simulink model "ReactionWheel"  (R2020a)
settings: Solver=FixedStepAuto  StartTime=0.0  StopTime=100  FixedStep=0.00005  RelTol=1e-3
libraries: simulink x8, aerolibconvert2 x2
settings Model: Creator=b_ant  LastModifiedBy=DELL

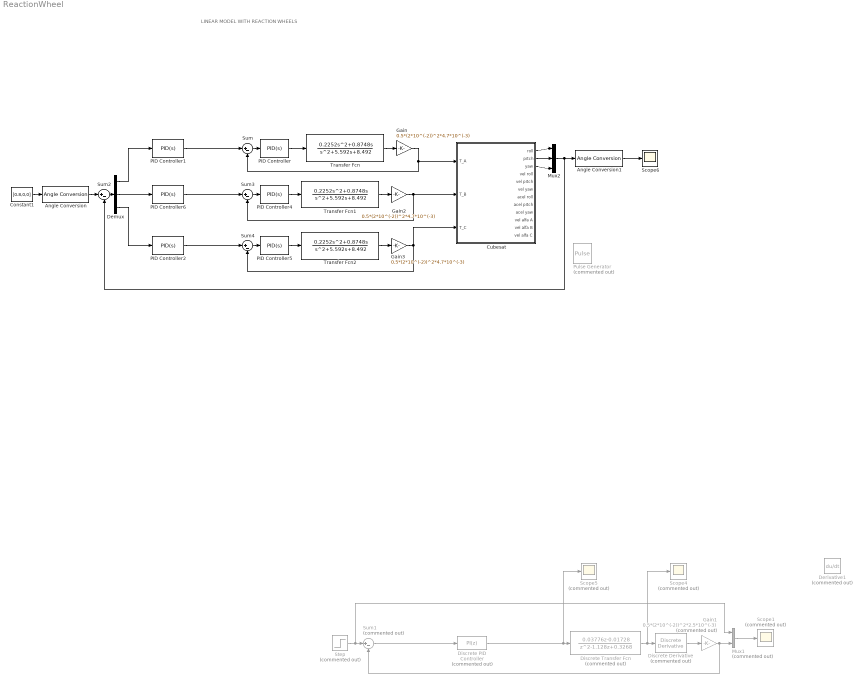
== system ReactionWheel ==
  note: LINEAR MODEL WITH REACTION WHEELS
  Angle Conversion : aerolibconvert2/Angle Conversion  IU=deg  OU=rad
  Angle Conversion1 : aerolibconvert2/Angle Conversion  IU=rad  OU=deg
  Constant1 : Constant  Value=[0.8,0,0]
  Cubesat : Subsystem  mask{Iw=9.4*10^-7, Ib=6.88*10^-4, mw=0.0047, lw=0.092, Bw=0}
      mask prompts: Iw "Momento de inercia de rueda de reacción"; Ib "Momento de inercia de CubeSat"; mw "Masa de Rueda de reacción"; lw "Longitud de CM de CubeSat a eje de rueda"; Bw "Coeficiente de friccion"
  Demux : Demux  Outputs=3
  Derivative1 : Derivative  Commented=on
  Discrete Transfer Fcn : DiscreteTransferFcn  Commented=on  Numerator=[0.03776 -0.01728]  Denominator=[1 -1.128 0.3268]
  Discrete Derivative : simulink/Discrete/Discrete Derivative  Commented=on  gainval=1  ICPrevScaledInput=0  OutMin=[]  OutMax=[]  OutDataType=fixdt(1, 16)  OutScaling=2^-10  DoSatur=off
  Discrete PID Controller : simulink/Continuous/PID Controller  Commented=on  Controller=PI  Form=Parallel  TimeDomain=Discrete-time  UseExternalTs=off  SampleTime=0.1  IntegratorMethod=Trapezoidal  FilterMethod=Forward Euler  ControllerParametersSource=internal  P=2275968.39507176  I=49240241.1330709  D=0  UseFilter=on  N=100  TunerSelectOption=Transfer Function Based (PID Tuner App)  InitialConditionSource=internal  InitialConditionForIntegrator=0  InitialConditionForFilter=0  DifferentiatorICPrevScaledInput=0  ExternalReset=none  TrackingMode=off  Kt=1  LimitOutput=on  UpperSaturationLimit=4999  LowerSaturationLimit=-4999  LinearizeAsGain=on  AntiWindupMode=none  Kb=1  POutMin=[]  POutMax=[]  IOutMin=[]  IOutMax=[]  DOutMin=[]  DOutMax=[]  NOutMin=[]  NOutMax=[]  SumOutMin=[]  SumOutMax=[]  SaturationOutMin=[]  SaturationOutMax=[]  PParamMin=[]  PParamMax=[]  IParamMin=[]  IParamMax=[]  DParamMin=[]  DParamMax=[]  NParamMin=[]  NParamMax=[]  KbParamMin=[]  KbParamMax=[]  KtParamMin=[]  KtParamMax=[]  KbOutMin=[]  KbOutMax=[]  KtOutMin=[]  KtOutMax=[]  IntegratorOutMin=[]  IntegratorOutMax=[]  FilterOutMin=[]  FilterOutMax=[]  SumI1OutMin=[]  SumI1OutMax=[]  SumI2OutMin=[]  SumI2OutMax=[]  SumI3OutMin=[]  SumI3OutMax=[]  SumI4OutMin=[]  SumI4OutMax=[]  SumDOutMin=[]  SumDOutMax=[]  DifferentiatorOutMin=[]  DifferentiatorOutMax=[]  FilterDiffOutCoefMin=[]  FilterDiffOutCoefMax=[]  ReciprocalOutMin=[]  ReciprocalOutMax=[]  SumDenOutMin=[]  SumDenOutMax=[]  SumNumOutMin=[]  SumNumOutMax=[]  DivideOutMin=[]  DivideOutMax=[]  UdiffTsProdOutMin=[]  UdiffTsProdOutMax=[]  NTsProdOutMin=[]  NTsProdOutMax=[]  UintegralTsProdOutMin=[]  UintegralTsProdOutMax=[]  UngainTsProdOutMin=[]  UngainTsProdOutMax=[]  IntegratorContinuousStateAttributes=''  IntegratorStateMustResolveToSignalObject=off  IntegratorRTWStateStorageClass=Auto  FilterContinuousStateAttributes=''  FilterStateMustResolveToSignalObject=off  FilterRTWStateStorageClass=Auto  ParallelPVariant=InternalParameters  IdealPVariant=Disabled  IVariant=InternalParameters  DVariant=Disabled  IntegratorVariant=Discrete  SatVariant=Enabled  AWVariant=Passthrough  PCopyVariant=Disabled  TRVariant=Disabled  FdbkBlocksVariant=Forward  IdealPFdbkVariant=Disabled  SatFdbkVariant=Disabled  DerivativeFilterVariant=Disabled  NVariant=Disabled  NCopyVariant=Disabled_SignalSpec  FilterICVariant=Disabled  IntegratorICVariant=InternalICs  ExternalResetVariant=Disabled  TRSumVariant=Passthrough  SumFdbkVariant=Disabled  SumVariant=Sum_PI  TsampFilterVariant=InternalTs  TsampNgainVariant=Passthrough  TsampIntegralVariant=Passthrough
  Gain : Gain  Gain=0.5*(2*10^(-2))^2*4.7*10^(-3)
  Gain1 : Gain  Commented=on  Gain=0.5*(2*10^(-2))^2*2.5*10^(-3)
  Gain2 : Gain  Gain=0.5*(2*10^(-2))^2*4.7*10^(-3)
  Gain3 : Gain  Gain=0.5*(2*10^(-2))^2*4.7*10^(-3)
  Mux1 : Mux  Commented=on  Inputs=2
  Mux2 : Mux  Inputs=3
  PID Controller : simulink/Continuous/PID Controller  Controller=PID  Form=Parallel  TimeDomain=Continuous-time  UseExternalTs=off  SampleTime=1  IntegratorMethod=Forward Euler  FilterMethod=Forward Euler  ControllerParametersSource=internal  P=0  I=15673894481.5576  D=0  UseFilter=on  N=100  TunerSelectOption=Transfer Function Based (PID Tuner App)  InitialConditionSource=internal  InitialConditionForIntegrator=0  InitialConditionForFilter=0  DifferentiatorICPrevScaledInput=0  ExternalReset=none  TrackingMode=off  Kt=1  LimitOutput=on  UpperSaturationLimit=4999  LowerSaturationLimit=-4999  LinearizeAsGain=on  AntiWindupMode=none  Kb=1  POutMin=[]  POutMax=[]  IOutMin=[]  IOutMax=[]  DOutMin=[]  DOutMax=[]  NOutMin=[]  NOutMax=[]  SumOutMin=[]  SumOutMax=[]  SaturationOutMin=[]  SaturationOutMax=[]  PParamMin=[]  PParamMax=[]  IParamMin=[]  IParamMax=[]  DParamMin=[]  DParamMax=[]  NParamMin=[]  NParamMax=[]  KbParamMin=[]  KbParamMax=[]  KtParamMin=[]  KtParamMax=[]  KbOutMin=[]  KbOutMax=[]  KtOutMin=[]  KtOutMax=[]  IntegratorOutMin=[]  IntegratorOutMax=[]  FilterOutMin=[]  FilterOutMax=[]  SumI1OutMin=[]  SumI1OutMax=[]  SumI2OutMin=[]  SumI2OutMax=[]  SumI3OutMin=[]  SumI3OutMax=[]  SumI4OutMin=[]  SumI4OutMax=[]  SumDOutMin=[]  SumDOutMax=[]  DifferentiatorOutMin=[]  DifferentiatorOutMax=[]  FilterDiffOutCoefMin=[]  FilterDiffOutCoefMax=[]  ReciprocalOutMin=[]  ReciprocalOutMax=[]  SumDenOutMin=[]  SumDenOutMax=[]  SumNumOutMin=[]  SumNumOutMax=[]  DivideOutMin=[]  DivideOutMax=[]  UdiffTsProdOutMin=[]  UdiffTsProdOutMax=[]  NTsProdOutMin=[]  NTsProdOutMax=[]  UintegralTsProdOutMin=[]  UintegralTsProdOutMax=[]  UngainTsProdOutMin=[]  UngainTsProdOutMax=[]  IntegratorContinuousStateAttributes=''  IntegratorStateMustResolveToSignalObject=off  IntegratorRTWStateStorageClass=Auto  FilterContinuousStateAttributes=''  FilterStateMustResolveToSignalObject=off  FilterRTWStateStorageClass=Auto  ParallelPVariant=InternalParameters  IdealPVariant=Disabled  IVariant=InternalParameters  DVariant=InternalParameters  IntegratorVariant=Continuous  SatVariant=Enabled  AWVariant=Passthrough  PCopyVariant=Disabled  TRVariant=Disabled  FdbkBlocksVariant=Forward  IdealPFdbkVariant=Disabled  SatFdbkVariant=Disabled  DerivativeFilterVariant=ContFilter  NVariant=InternalParameters  NCopyVariant=Disabled  FilterICVariant=InternalICsFilter  IntegratorICVariant=InternalICs  ExternalResetVariant=Disabled  TRSumVariant=Passthrough  SumFdbkVariant=Disabled  SumVariant=Sum_PID  TsampFilterVariant=InternalTs  TsampNgainVariant=Passthrough  TsampIntegralVariant=Passthrough
  PID Controller1 : simulink/Continuous/PID Controller  Controller=PID  Form=Parallel  TimeDomain=Continuous-time  UseExternalTs=off  SampleTime=-1  IntegratorMethod=Forward Euler  FilterMethod=Forward Euler  ControllerParametersSource=internal  P=-3.24987577526797e-07  I=-2.1955547593358e-10  D=-8.46467148788469e-05  UseFilter=on  N=11.428279760416  TunerSelectOption=Transfer Function Based (PID Tuner App)  InitialConditionSource=internal  InitialConditionForIntegrator=0  InitialConditionForFilter=0  DifferentiatorICPrevScaledInput=0  ExternalReset=none  TrackingMode=off  Kt=1  LimitOutput=off  UpperSaturationLimit=3*10^(-3)  LowerSaturationLimit=-3*10^(-3)  LinearizeAsGain=on  AntiWindupMode=none  Kb=1  POutMin=[]  POutMax=[]  IOutMin=[]  IOutMax=[]  DOutMin=[]  DOutMax=[]  NOutMin=[]  NOutMax=[]  SumOutMin=[]  SumOutMax=[]  SaturationOutMin=[]  SaturationOutMax=[]  PParamMin=[]  PParamMax=[]  IParamMin=[]  IParamMax=[]  DParamMin=[]  DParamMax=[]  NParamMin=[]  NParamMax=[]  KbParamMin=[]  KbParamMax=[]  KtParamMin=[]  KtParamMax=[]  KbOutMin=[]  KbOutMax=[]  KtOutMin=[]  KtOutMax=[]  IntegratorOutMin=[]  IntegratorOutMax=[]  FilterOutMin=[]  FilterOutMax=[]  SumI1OutMin=[]  SumI1OutMax=[]  SumI2OutMin=[]  SumI2OutMax=[]  SumI3OutMin=[]  SumI3OutMax=[]  SumI4OutMin=[]  SumI4OutMax=[]  SumDOutMin=[]  SumDOutMax=[]  DifferentiatorOutMin=[]  DifferentiatorOutMax=[]  FilterDiffOutCoefMin=[]  FilterDiffOutCoefMax=[]  ReciprocalOutMin=[]  ReciprocalOutMax=[]  SumDenOutMin=[]  SumDenOutMax=[]  SumNumOutMin=[]  SumNumOutMax=[]  DivideOutMin=[]  DivideOutMax=[]  UdiffTsProdOutMin=[]  UdiffTsProdOutMax=[]  NTsProdOutMin=[]  NTsProdOutMax=[]  UintegralTsProdOutMin=[]  UintegralTsProdOutMax=[]  UngainTsProdOutMin=[]  UngainTsProdOutMax=[]  IntegratorContinuousStateAttributes=''  IntegratorStateMustResolveToSignalObject=off  IntegratorRTWStateStorageClass=Auto  FilterContinuousStateAttributes=''  FilterStateMustResolveToSignalObject=off  FilterRTWStateStorageClass=Auto  ParallelPVariant=InternalParameters  IdealPVariant=Disabled  IVariant=InternalParameters  DVariant=InternalParameters  IntegratorVariant=Continuous  SatVariant=Disabled  AWVariant=Passthrough  PCopyVariant=Disabled  TRVariant=Disabled  FdbkBlocksVariant=Forward  IdealPFdbkVariant=Disabled  SatFdbkVariant=Disabled  DerivativeFilterVariant=ContFilter  NVariant=InternalParameters  NCopyVariant=Disabled  FilterICVariant=InternalICsFilter  IntegratorICVariant=InternalICs  ExternalResetVariant=Disabled  TRSumVariant=Passthrough  SumFdbkVariant=Disabled  SumVariant=Sum_PID  TsampFilterVariant=InternalTs  TsampNgainVariant=Passthrough  TsampIntegralVariant=Passthrough
  PID Controller2 : simulink/Continuous/PID Controller  Controller=PID  Form=Parallel  TimeDomain=Continuous-time  UseExternalTs=off  SampleTime=-1  IntegratorMethod=Forward Euler  FilterMethod=Forward Euler  ControllerParametersSource=internal  P=-3.24987577526797e-07  I=-2.1955547593358e-10  D=-8.46467148788469e-05  UseFilter=on  N=11.428279760416  TunerSelectOption=Transfer Function Based (PID Tuner App)  InitialConditionSource=internal  InitialConditionForIntegrator=0  InitialConditionForFilter=0  DifferentiatorICPrevScaledInput=0  ExternalReset=none  TrackingMode=off  Kt=1  LimitOutput=off  UpperSaturationLimit=3*10^(-3)  LowerSaturationLimit=-3*10^(-3)  LinearizeAsGain=on  AntiWindupMode=none  Kb=1  POutMin=[]  POutMax=[]  IOutMin=[]  IOutMax=[]  DOutMin=[]  DOutMax=[]  NOutMin=[]  NOutMax=[]  SumOutMin=[]  SumOutMax=[]  SaturationOutMin=[]  SaturationOutMax=[]  PParamMin=[]  PParamMax=[]  IParamMin=[]  IParamMax=[]  DParamMin=[]  DParamMax=[]  NParamMin=[]  NParamMax=[]  KbParamMin=[]  KbParamMax=[]  KtParamMin=[]  KtParamMax=[]  KbOutMin=[]  KbOutMax=[]  KtOutMin=[]  KtOutMax=[]  IntegratorOutMin=[]  IntegratorOutMax=[]  FilterOutMin=[]  FilterOutMax=[]  SumI1OutMin=[]  SumI1OutMax=[]  SumI2OutMin=[]  SumI2OutMax=[]  SumI3OutMin=[]  SumI3OutMax=[]  SumI4OutMin=[]  SumI4OutMax=[]  SumDOutMin=[]  SumDOutMax=[]  DifferentiatorOutMin=[]  DifferentiatorOutMax=[]  FilterDiffOutCoefMin=[]  FilterDiffOutCoefMax=[]  ReciprocalOutMin=[]  ReciprocalOutMax=[]  SumDenOutMin=[]  SumDenOutMax=[]  SumNumOutMin=[]  SumNumOutMax=[]  DivideOutMin=[]  DivideOutMax=[]  UdiffTsProdOutMin=[]  UdiffTsProdOutMax=[]  NTsProdOutMin=[]  NTsProdOutMax=[]  UintegralTsProdOutMin=[]  UintegralTsProdOutMax=[]  UngainTsProdOutMin=[]  UngainTsProdOutMax=[]  IntegratorContinuousStateAttributes=''  IntegratorStateMustResolveToSignalObject=off  IntegratorRTWStateStorageClass=Auto  FilterContinuousStateAttributes=''  FilterStateMustResolveToSignalObject=off  FilterRTWStateStorageClass=Auto  ParallelPVariant=InternalParameters  IdealPVariant=Disabled  IVariant=InternalParameters  DVariant=InternalParameters  IntegratorVariant=Continuous  SatVariant=Disabled  AWVariant=Passthrough  PCopyVariant=Disabled  TRVariant=Disabled  FdbkBlocksVariant=Forward  IdealPFdbkVariant=Disabled  SatFdbkVariant=Disabled  DerivativeFilterVariant=ContFilter  NVariant=InternalParameters  NCopyVariant=Disabled  FilterICVariant=InternalICsFilter  IntegratorICVariant=InternalICs  ExternalResetVariant=Disabled  TRSumVariant=Passthrough  SumFdbkVariant=Disabled  SumVariant=Sum_PID  TsampFilterVariant=InternalTs  TsampNgainVariant=Passthrough  TsampIntegralVariant=Passthrough
  PID Controller4 : simulink/Continuous/PID Controller  Controller=PID  Form=Parallel  TimeDomain=Continuous-time  UseExternalTs=off  SampleTime=1  IntegratorMethod=Forward Euler  FilterMethod=Forward Euler  ControllerParametersSource=internal  P=0  I=15673894481.5576  D=0  UseFilter=on  N=100  TunerSelectOption=Transfer Function Based (PID Tuner App)  InitialConditionSource=internal  InitialConditionForIntegrator=0  InitialConditionForFilter=0  DifferentiatorICPrevScaledInput=0  ExternalReset=none  TrackingMode=off  Kt=1  LimitOutput=on  UpperSaturationLimit=4999  LowerSaturationLimit=-4999  LinearizeAsGain=on  AntiWindupMode=none  Kb=1  POutMin=[]  POutMax=[]  IOutMin=[]  IOutMax=[]  DOutMin=[]  DOutMax=[]  NOutMin=[]  NOutMax=[]  SumOutMin=[]  SumOutMax=[]  SaturationOutMin=[]  SaturationOutMax=[]  PParamMin=[]  PParamMax=[]  IParamMin=[]  IParamMax=[]  DParamMin=[]  DParamMax=[]  NParamMin=[]  NParamMax=[]  KbParamMin=[]  KbParamMax=[]  KtParamMin=[]  KtParamMax=[]  KbOutMin=[]  KbOutMax=[]  KtOutMin=[]  KtOutMax=[]  IntegratorOutMin=[]  IntegratorOutMax=[]  FilterOutMin=[]  FilterOutMax=[]  SumI1OutMin=[]  SumI1OutMax=[]  SumI2OutMin=[]  SumI2OutMax=[]  SumI3OutMin=[]  SumI3OutMax=[]  SumI4OutMin=[]  SumI4OutMax=[]  SumDOutMin=[]  SumDOutMax=[]  DifferentiatorOutMin=[]  DifferentiatorOutMax=[]  FilterDiffOutCoefMin=[]  FilterDiffOutCoefMax=[]  ReciprocalOutMin=[]  ReciprocalOutMax=[]  SumDenOutMin=[]  SumDenOutMax=[]  SumNumOutMin=[]  SumNumOutMax=[]  DivideOutMin=[]  DivideOutMax=[]  UdiffTsProdOutMin=[]  UdiffTsProdOutMax=[]  NTsProdOutMin=[]  NTsProdOutMax=[]  UintegralTsProdOutMin=[]  UintegralTsProdOutMax=[]  UngainTsProdOutMin=[]  UngainTsProdOutMax=[]  IntegratorContinuousStateAttributes=''  IntegratorStateMustResolveToSignalObject=off  IntegratorRTWStateStorageClass=Auto  FilterContinuousStateAttributes=''  FilterStateMustResolveToSignalObject=off  FilterRTWStateStorageClass=Auto  ParallelPVariant=InternalParameters  IdealPVariant=Disabled  IVariant=InternalParameters  DVariant=InternalParameters  IntegratorVariant=Continuous  SatVariant=Enabled  AWVariant=Passthrough  PCopyVariant=Disabled  TRVariant=Disabled  FdbkBlocksVariant=Forward  IdealPFdbkVariant=Disabled  SatFdbkVariant=Disabled  DerivativeFilterVariant=ContFilter  NVariant=InternalParameters  NCopyVariant=Disabled  FilterICVariant=InternalICsFilter  IntegratorICVariant=InternalICs  ExternalResetVariant=Disabled  TRSumVariant=Passthrough  SumFdbkVariant=Disabled  SumVariant=Sum_PID  TsampFilterVariant=InternalTs  TsampNgainVariant=Passthrough  TsampIntegralVariant=Passthrough
  PID Controller5 : simulink/Continuous/PID Controller  Controller=PID  Form=Parallel  TimeDomain=Continuous-time  UseExternalTs=off  SampleTime=1  IntegratorMethod=Forward Euler  FilterMethod=Forward Euler  ControllerParametersSource=internal  P=0  I=15673894481.5576  D=0  UseFilter=on  N=100  TunerSelectOption=Transfer Function Based (PID Tuner App)  InitialConditionSource=internal  InitialConditionForIntegrator=0  InitialConditionForFilter=0  DifferentiatorICPrevScaledInput=0  ExternalReset=none  TrackingMode=off  Kt=1  LimitOutput=on  UpperSaturationLimit=4999  LowerSaturationLimit=-4999  LinearizeAsGain=on  AntiWindupMode=none  Kb=1  POutMin=[]  POutMax=[]  IOutMin=[]  IOutMax=[]  DOutMin=[]  DOutMax=[]  NOutMin=[]  NOutMax=[]  SumOutMin=[]  SumOutMax=[]  SaturationOutMin=[]  SaturationOutMax=[]  PParamMin=[]  PParamMax=[]  IParamMin=[]  IParamMax=[]  DParamMin=[]  DParamMax=[]  NParamMin=[]  NParamMax=[]  KbParamMin=[]  KbParamMax=[]  KtParamMin=[]  KtParamMax=[]  KbOutMin=[]  KbOutMax=[]  KtOutMin=[]  KtOutMax=[]  IntegratorOutMin=[]  IntegratorOutMax=[]  FilterOutMin=[]  FilterOutMax=[]  SumI1OutMin=[]  SumI1OutMax=[]  SumI2OutMin=[]  SumI2OutMax=[]  SumI3OutMin=[]  SumI3OutMax=[]  SumI4OutMin=[]  SumI4OutMax=[]  SumDOutMin=[]  SumDOutMax=[]  DifferentiatorOutMin=[]  DifferentiatorOutMax=[]  FilterDiffOutCoefMin=[]  FilterDiffOutCoefMax=[]  ReciprocalOutMin=[]  ReciprocalOutMax=[]  SumDenOutMin=[]  SumDenOutMax=[]  SumNumOutMin=[]  SumNumOutMax=[]  DivideOutMin=[]  DivideOutMax=[]  UdiffTsProdOutMin=[]  UdiffTsProdOutMax=[]  NTsProdOutMin=[]  NTsProdOutMax=[]  UintegralTsProdOutMin=[]  UintegralTsProdOutMax=[]  UngainTsProdOutMin=[]  UngainTsProdOutMax=[]  IntegratorContinuousStateAttributes=''  IntegratorStateMustResolveToSignalObject=off  IntegratorRTWStateStorageClass=Auto  FilterContinuousStateAttributes=''  FilterStateMustResolveToSignalObject=off  FilterRTWStateStorageClass=Auto  ParallelPVariant=InternalParameters  IdealPVariant=Disabled  IVariant=InternalParameters  DVariant=InternalParameters  IntegratorVariant=Continuous  SatVariant=Enabled  AWVariant=Passthrough  PCopyVariant=Disabled  TRVariant=Disabled  FdbkBlocksVariant=Forward  IdealPFdbkVariant=Disabled  SatFdbkVariant=Disabled  DerivativeFilterVariant=ContFilter  NVariant=InternalParameters  NCopyVariant=Disabled  FilterICVariant=InternalICsFilter  IntegratorICVariant=InternalICs  ExternalResetVariant=Disabled  TRSumVariant=Passthrough  SumFdbkVariant=Disabled  SumVariant=Sum_PID  TsampFilterVariant=InternalTs  TsampNgainVariant=Passthrough  TsampIntegralVariant=Passthrough
  PID Controller6 : simulink/Continuous/PID Controller  Controller=PID  Form=Parallel  TimeDomain=Continuous-time  UseExternalTs=off  SampleTime=-1  IntegratorMethod=Forward Euler  FilterMethod=Forward Euler  ControllerParametersSource=internal  P=-3.24987577526797e-07  I=-2.1955547593358e-10  D=-8.46467148788469e-05  UseFilter=on  N=11.428279760416  TunerSelectOption=Transfer Function Based (PID Tuner App)  InitialConditionSource=internal  InitialConditionForIntegrator=0  InitialConditionForFilter=0  DifferentiatorICPrevScaledInput=0  ExternalReset=none  TrackingMode=off  Kt=1  LimitOutput=off  UpperSaturationLimit=3*10^(-3)  LowerSaturationLimit=-3*10^(-3)  LinearizeAsGain=on  AntiWindupMode=none  Kb=1  POutMin=[]  POutMax=[]  IOutMin=[]  IOutMax=[]  DOutMin=[]  DOutMax=[]  NOutMin=[]  NOutMax=[]  SumOutMin=[]  SumOutMax=[]  SaturationOutMin=[]  SaturationOutMax=[]  PParamMin=[]  PParamMax=[]  IParamMin=[]  IParamMax=[]  DParamMin=[]  DParamMax=[]  NParamMin=[]  NParamMax=[]  KbParamMin=[]  KbParamMax=[]  KtParamMin=[]  KtParamMax=[]  KbOutMin=[]  KbOutMax=[]  KtOutMin=[]  KtOutMax=[]  IntegratorOutMin=[]  IntegratorOutMax=[]  FilterOutMin=[]  FilterOutMax=[]  SumI1OutMin=[]  SumI1OutMax=[]  SumI2OutMin=[]  SumI2OutMax=[]  SumI3OutMin=[]  SumI3OutMax=[]  SumI4OutMin=[]  SumI4OutMax=[]  SumDOutMin=[]  SumDOutMax=[]  DifferentiatorOutMin=[]  DifferentiatorOutMax=[]  FilterDiffOutCoefMin=[]  FilterDiffOutCoefMax=[]  ReciprocalOutMin=[]  ReciprocalOutMax=[]  SumDenOutMin=[]  SumDenOutMax=[]  SumNumOutMin=[]  SumNumOutMax=[]  DivideOutMin=[]  DivideOutMax=[]  UdiffTsProdOutMin=[]  UdiffTsProdOutMax=[]  NTsProdOutMin=[]  NTsProdOutMax=[]  UintegralTsProdOutMin=[]  UintegralTsProdOutMax=[]  UngainTsProdOutMin=[]  UngainTsProdOutMax=[]  IntegratorContinuousStateAttributes=''  IntegratorStateMustResolveToSignalObject=off  IntegratorRTWStateStorageClass=Auto  FilterContinuousStateAttributes=''  FilterStateMustResolveToSignalObject=off  FilterRTWStateStorageClass=Auto  ParallelPVariant=InternalParameters  IdealPVariant=Disabled  IVariant=InternalParameters  DVariant=InternalParameters  IntegratorVariant=Continuous  SatVariant=Disabled  AWVariant=Passthrough  PCopyVariant=Disabled  TRVariant=Disabled  FdbkBlocksVariant=Forward  IdealPFdbkVariant=Disabled  SatFdbkVariant=Disabled  DerivativeFilterVariant=ContFilter  NVariant=InternalParameters  NCopyVariant=Disabled  FilterICVariant=InternalICsFilter  IntegratorICVariant=InternalICs  ExternalResetVariant=Disabled  TRSumVariant=Passthrough  SumFdbkVariant=Disabled  SumVariant=Sum_PID  TsampFilterVariant=InternalTs  TsampNgainVariant=Passthrough  TsampIntegralVariant=Passthrough
  Pulse Generator : DiscretePulseGenerator  Commented=on  PulseType=Time based  Amplitude=1*10^(-4)  Period=7  PulseWidth=50
  Scope1 : Scope  Commented=on
  Scope4 : Scope  Commented=on
  Scope5 : Scope  Commented=on
  Scope6 : Scope
  Step : Step  Commented=on  After=1*10^(-4)  SampleTime=0
  Sum{,2..4} (4 alike) : Sum  Inputs=|+-
  Sum1 : Sum  Commented=on  Inputs=|+-
  Transfer Fcn : TransferFcn  Numerator=[0.2252 0.8748 0]  Denominator=[1 5.592 8.492]
  Transfer Fcn1 : TransferFcn  Numerator=[0.2252 0.8748 0]  Denominator=[1 5.592 8.492]
  Transfer Fcn2 : TransferFcn  Numerator=[0.2252 0.8748 0]  Denominator=[1 5.592 8.492]
  wires:
  Discrete Derivative/1 -> Gain1/1
  Gain1/1 -> Mux1/2, Sum1/2
  Mux1/1 -> Scope1/1
  Step/1 -> Mux1/1, Sum1/1
  Discrete Transfer Fcn/1 -> Scope4/1, Discrete Derivative/1
  Discrete PID Controller/1 -> Scope5/1, Discrete Transfer Fcn/1
  Sum1/1 -> Discrete PID Controller/1
  Mux2/1 -> Angle Conversion1/1, Sum2/2
  Demux/3 -> PID Controller2/1
  Cubesat/2(pitch) -> Mux2/2
  Cubesat/1(roll) -> Mux2/1
  Cubesat/3(yaw) -> Mux2/3
  Sum2/1 -> Demux/1
  Demux/1 -> PID Controller1/1
  Constant1/1 -> Angle Conversion/1
  Angle Conversion/1 -> Sum2/1
  Demux/2 -> PID Controller6/1
  Angle Conversion1/1 -> Scope6/1
  PID Controller6/1 -> Sum3/1
  PID Controller2/1 -> Sum4/1
  Gain3/1 -> Cubesat/3(T_C), Sum4/2
  Transfer Fcn1/1 -> Gain2/1
  Sum4/1 -> PID Controller5/1
  PID Controller5/1 -> Transfer Fcn2/1
  PID Controller1/1 -> Sum/1
  PID Controller4/1 -> Transfer Fcn1/1
  Transfer Fcn2/1 -> Gain3/1
  Sum/1 -> PID Controller/1
  Transfer Fcn/1 -> Gain/1
  Sum3/1 -> PID Controller4/1
  Gain2/1 -> Cubesat/2(T_B), Sum3/2
  PID Controller/1 -> Transfer Fcn/1
  Gain/1 -> Cubesat/1(T_A), Sum/2

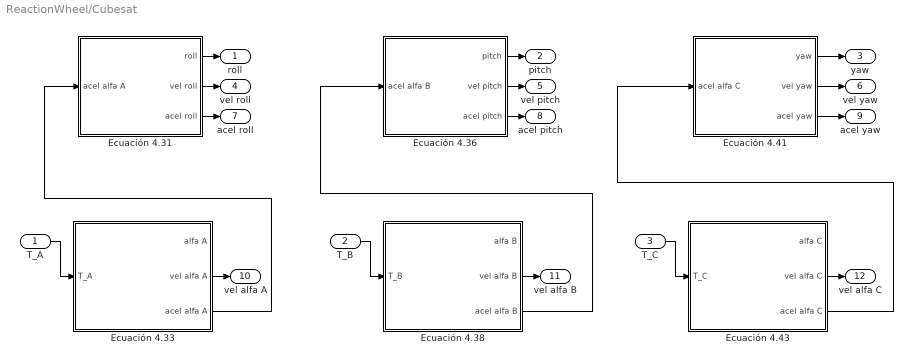
== system ReactionWheel/Cubesat ==
  T_A : Inport
  T_B : Inport  Port=2
  T_C : Inport  Port=3
  Ecuación 4.31 : Subsystem
  Ecuación 4.33 : Subsystem
  Ecuación 4.36 : Subsystem
  Ecuación 4.38 : Subsystem
  Ecuación 4.41 : Subsystem
  Ecuación 4.43 : Subsystem
  roll : Outport
  pitch : Outport  Port=2
  yaw : Outport  Port=3
  vel roll : Outport  Port=4
  vel pitch : Outport  Port=5
  vel yaw : Outport  Port=6
  acel roll : Outport  Port=7
  acel pitch : Outport  Port=8
  acel yaw : Outport  Port=9
  vel alfa A : Outport  Port=10
  vel alfa B : Outport  Port=11
  vel alfa C : Outport  Port=12
  wires:
  Ecuación 4.41/2(vel yaw) -> vel yaw/1
  Ecuación 4.41/3(acel yaw) -> acel yaw/1
  Ecuación 4.41/1(yaw) -> yaw/1
  Ecuación 4.33/3(acel alfa A) -> Ecuación 4.31/1(acel alfa A)
  Ecuación 4.43/3(acel alfa C) -> Ecuación 4.41/1(acel alfa C)
  Ecuación 4.33/2(vel alfa A) -> vel alfa A/1
  Ecuación 4.36/2(vel pitch) -> vel pitch/1
  T_B/1 -> Ecuación 4.38/1(T_B)
  T_A/1 -> Ecuación 4.33/1(T_A)
  Ecuación 4.43/2(vel alfa C) -> vel alfa C/1
  Ecuación 4.31/1(roll) -> roll/1
  Ecuación 4.36/1(pitch) -> pitch/1
  Ecuación 4.31/2(vel roll) -> vel roll/1
  Ecuación 4.31/3(acel roll) -> acel roll/1
  Ecuación 4.38/2(vel alfa B) -> vel alfa B/1
  Ecuación 4.36/3(acel pitch) -> acel pitch/1
  T_C/1 -> Ecuación 4.43/1(T_C)
  Ecuación 4.38/3(acel alfa B) -> Ecuación 4.36/1(acel alfa B)

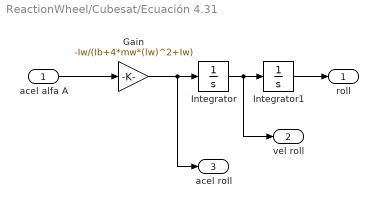
== system ReactionWheel/Cubesat/Ecuación 4.31 ==
  acel alfa A : Inport
  Gain : Gain  Gain=-Iw/(Ib+4*mw*(lw)^2+Iw)
  Integrator : Integrator
  Integrator1 : Integrator
  roll : Outport
  vel roll : Outport  Port=2
  acel roll : Outport  Port=3
  wires:
  acel alfa A/1 -> Gain/1
  Gain/1 -> acel roll/1, Integrator/1
  Integrator/1 -> vel roll/1, Integrator1/1
  Integrator1/1 -> roll/1

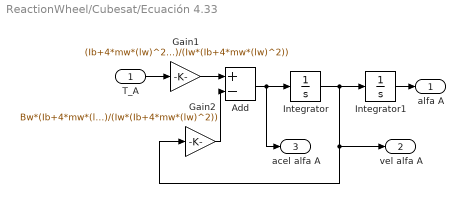
== system ReactionWheel/Cubesat/Ecuación 4.33 ==
  T_A : Inport
  Add : Sum  Inputs=+-
  Gain1 : Gain  Gain=(Ib+4*mw*(lw)^2+Iw)/(Iw*(Ib+4*mw*(lw)^2))
  Gain2 : Gain  Gain=Bw*(Ib+4*mw*(lw)^2+Iw)/(Iw*(Ib+4*mw*(lw)^2))
  Integrator : Integrator
  Integrator1 : Integrator
  alfa A : Outport
  vel alfa A : Outport  Port=2
  acel alfa A : Outport  Port=3
  wires:
  Integrator/1 -> Integrator1/1, vel alfa A/1, Gain2/1
  T_A/1 -> Gain1/1
  Gain2/1 -> Add/2
  Add/1 -> Integrator/1, acel alfa A/1
  Gain1/1 -> Add/1
  Integrator1/1 -> alfa A/1

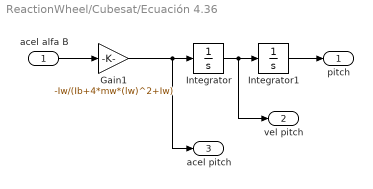
== system ReactionWheel/Cubesat/Ecuación 4.36 ==
  acel alfa B : Inport
  Gain1 : Gain  Gain=-Iw/(Ib+4*mw*(lw)^2+Iw)
  Integrator : Integrator
  Integrator1 : Integrator
  pitch : Outport
  vel pitch : Outport  Port=2
  acel pitch : Outport  Port=3
  wires:
  Gain1/1 -> acel pitch/1, Integrator/1
  Integrator/1 -> vel pitch/1, Integrator1/1
  acel alfa B/1 -> Gain1/1
  Integrator1/1 -> pitch/1

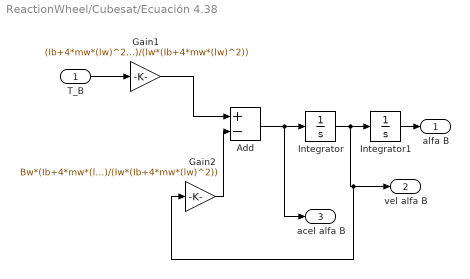
== system ReactionWheel/Cubesat/Ecuación 4.38 ==
  T_B : Inport
  Add : Sum  Inputs=+-
  Gain1 : Gain  Gain=(Ib+4*mw*(lw)^2+Iw)/(Iw*(Ib+4*mw*(lw)^2))
  Gain2 : Gain  Gain=Bw*(Ib+4*mw*(lw)^2+Iw)/(Iw*(Ib+4*mw*(lw)^2))
  Integrator : Integrator
  Integrator1 : Integrator
  alfa B : Outport
  vel alfa B : Outport  Port=2
  acel alfa B : Outport  Port=3
  wires:
  Integrator/1 -> Gain2/1, vel alfa B/1, Integrator1/1
  T_B/1 -> Gain1/1
  Gain2/1 -> Add/2
  Add/1 -> acel alfa B/1, Integrator/1
  Gain1/1 -> Add/1
  Integrator1/1 -> alfa B/1

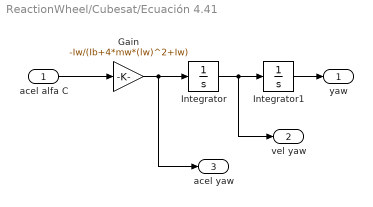
== system ReactionWheel/Cubesat/Ecuación 4.41 ==
  acel alfa C : Inport
  Gain : Gain  Gain=-Iw/(Ib+4*mw*(lw)^2+Iw)
  Integrator : Integrator
  Integrator1 : Integrator
  yaw : Outport
  vel yaw : Outport  Port=2
  acel yaw : Outport  Port=3
  wires:
  Gain/1 -> Integrator/1, acel yaw/1
  Integrator/1 -> Integrator1/1, vel yaw/1
  acel alfa C/1 -> Gain/1
  Integrator1/1 -> yaw/1

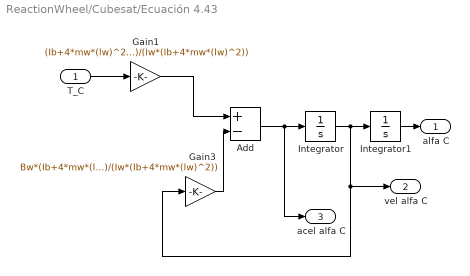
== system ReactionWheel/Cubesat/Ecuación 4.43 ==
  T_C : Inport
  Add : Sum  Inputs=+-
  Gain1 : Gain  Gain=(Ib+4*mw*(lw)^2+Iw)/(Iw*(Ib+4*mw*(lw)^2))
  Gain3 : Gain  Gain=Bw*(Ib+4*mw*(lw)^2+Iw)/(Iw*(Ib+4*mw*(lw)^2))
  Integrator : Integrator
  Integrator1 : Integrator
  alfa C : Outport
  vel alfa C : Outport  Port=2
  acel alfa C : Outport  Port=3
  wires:
  T_C/1 -> Gain1/1
  Gain3/1 -> Add/2
  Add/1 -> acel alfa C/1, Integrator/1
  Gain1/1 -> Add/1
  Integrator1/1 -> alfa C/1
  Integrator/1 -> Gain3/1, vel alfa C/1, Integrator1/1
